simulink model "simulation_file"  (R2023b)
settings: Solver=FixedStepAuto  StartTime=0.0  StopTime=16  FixedStep=0.001  RelTol=1e-3
InitFcn:
  | importfrankaEmikaPanda
values from neighbouring files (symbols this model uses):
  d_influence = 0.06    [distance_with_linesegments_test.m]    (also in importfrankaEmikaPanda.m; matlab_obstacle_avoidance.m = 0.04)
  d_stop = 0.02    [distance_with_linesegments_test.m]    (also in importfrankaEmikaPanda.m; matlab_obstacle_avoidance.m = 0.01)
  Gripper_orientation = [-pi/4 0 0]    [importfrankaEmikaPanda.m]
  Gripper_position = [0 0 0.103399]    [importfrankaEmikaPanda.m]
  Homejointpositions = [0 ,0, 0, -pi/2, 0, pi/2, pi/4]    [importfrankaEmikaPanda.m]
  jointMaxValues = [2.8973, 1.7628, 2.8973, -0.0698, 2.8973, 3.7525, 2.8973]    [importfrankaEmikaPanda.m]
  jointMinValues = [-2.8973, -1.7628, -2.8973, -3.0718, -2.8973, 0.6500, -2.8973]    [importfrankaEmikaPanda.m]
  jointvelMaxValues = [2.1750 2.1750 2.1750 2.1750 2.6100 2.6100 2.6100]    [importfrankaEmikaPanda.m]
  jointvelMinValues = [-2.1750 -2.1750 -2.1750 -2.1750 -2.6100 -2.6100 -2.6100]    [importfrankaEmikaPanda.m]
  m = sqrt(det(JJt))    [computeManipulabilityJacobian.m]
  maxWaypoints = 20    [createWaypointData.m]    (also in importfrankaEmikaPanda.m)
  mdhparams = [ ... (first row only)    [importfrankaEmikaPanda.m]
  obstacle_sphere_1 = struct(     'type', OBSTACLE_SPHERE,      'center', [0, 0.20, 0.8],      'dimensions', [0.1, 0.1, 0.1],      'orientation', [1, 0, 0, 0],      'axis', 0  )    [importfrankaEmikaPanda.m]    (also in matlab_obstacle_avoidance.m = struct(     'type', OBSTACLE_SPHERE,      'center', [0.5545,)
  orientations = [0     0    0 ... (first row only)    [createWaypointData.m]    (also in importfrankaEmikaPanda.m = orientations'; matlab_obstacle_avoidance.m = orientations')
  ts = 0.01    [createWaypointData.m]    (also in importfrankaEmikaPanda.m = 0.001; matlab_obstacle_avoidance.m = 0.001)
  waypointAccels = zeros(size(waypointVels))    [createWaypointData.m]    (also in importfrankaEmikaPanda.m; matlab_obstacle_avoidance.m)
  waypoints = toolPositionHome' +              [0 0 0 ; 0 0 0 ; 0 0 0 ; 0 0 0 ; 0 0 0]'    [createWaypointData.m]    (also in importfrankaEmikaPanda.m = waypoints'; matlab_obstacle_avoidance.m = waypoints')
  waypointTimes = 0:4:16    [createWaypointData.m]    (also in importfrankaEmikaPanda.m; matlab_obstacle_avoidance.m)
  waypointVels = 0.1 *[ 0  0  0 ... (first row only)    [createWaypointData.m]    (also in importfrankaEmikaPanda.m; matlab_obstacle_avoidance.m)
  X = X + v0(1)    [plotCylinder.m]    (also in plotCylinder_foranimation.m)
  Y = Y + v0(2)    [plotCylinder.m]    (also in plotCylinder_foranimation.m)
  Z = Z + v0(3)    [plotCylinder.m]    (also in plotCylinder_foranimation.m)
undefined symbols (not defined in the file or in its folder): diff
libraries: sm_lib x98, nesl_utility x15, robotmaniplib x11, trajExampleUtils x9, robotcorelib x7
(part 3 of 4)

== system simulation_file/Franka Emika Panda/Franka_Robot/panda_link7 ==
  Inertia : sm_lib/Body Elements/Inertia  InertiaType=Custom  Mass=0  MassUnits=kg  CenterOfMass=[0, 0, 0]  CenterOfMassUnits=m  MomentsOfInertia=[0, 0, 0]  MomentsOfInertiaUnits=kg*m^2  ProductsOfInertia=[0, 0, 0]  ProductsOfInertiaUnits=kg*m^2  GraphicType=None  MarkerShape=Inertia  MarkerSize=20  GraphicVisPropType=SimpleVisualProperties  GraphicDiffuseColor=[0.5 0.5 0.5]  GraphicSpecularColor=[0.5 0.5 0.5 1.0]  GraphicAmbientColor=[0.15 0.15 0.15 1.0]  GraphicEmissiveColor=[0.0 0.0 0.0 1.0]  GraphicShininess=75  GraphicOpacity=1.0
  InertiaOriginTransform : sm_lib/Frames and Transforms/Rigid Transform  TranslationMethod=Cartesian  TranslationStandardOffset=0  TranslationStandardOffsetUnits=m  TranslationStandardAxis=+Z  TranslationCartesianOffset=[0, 0, 0]  TranslationCartesianOffsetUnits=m  TranslationROffset=0  TranslationROffsetUnits=m  TranslationZOffset=0  TranslationZOffsetUnits=m  TranslationThetaOffset=0  TranslationThetaOffsetUnits=deg  RotationMethod=RotationSequence  RotationAngleUnits=deg  RotationStandardAxis=+Z  RotationAngle=0.0  RotationArbitraryAxis=[0 0 1]  FollAlignAxisA=+X  BaseAlignAxisA=+Y  FollAlignAxisB=+Y  BaseAlignAxisB=+Z  RotationSequenceAxes=BaseAxes  RotationSequence=XYZ  RotationSequenceAngles=[0, 0, 0]  RotationSequenceAnglesUnits=rad  RotationMatrix=[1 0 0; 0 1 0; 0 0 1]  Quaternion=[1 0 0 0]
  ReferenceFrame : sm_lib/Frames and Transforms/Reference Frame
  Visual : sm_lib/Body Elements/File Solid  ExtGeomFileName=/home/shobhit/Documents/MATLAB/SupportPackages/R2023b/toolbox/robotics/supportpackages/robotlibrary/Robots/franka_description/meshes/visual/link7.stl  UnitType=Custom  ExtGeomFileUnits=m  StepReaderType=HEX  ExportConvexHullGeometry=off  InertiaType=Custom  Mass=0  MassUnits=kg  CenterOfMass=[0, 0, 0]  CenterOfMassUnits=m  MomentsOfInertia=[0, 0, 0]  MomentsOfInertiaUnits=kg*m^2  ProductsOfInertia=[0, 0, 0]  ProductsOfInertiaUnits=kg*m^2  BasedOnType=DensityFromFile  Density=1000  DensityUnits=kg/m^3  DoExposeReferenceFrame=on  SerializedFrames=<Frames/>  GraphicType=FromGeometry  MarkerShape=Sphere  MarkerSize=10  GraphicVisPropType=SimpleVisualProperties  GraphicDiffuseColor=[0.5, 0.5, 0.5]  GraphicSpecularColor=[0.5 0.5 0.5 1.0]  GraphicAmbientColor=[0.15 0.15 0.15 1.0]  GraphicEmissiveColor=[0.0 0.0 0.0 1.0]  GraphicShininess=75  GraphicOpacity=1
  VisualOriginTransform : sm_lib/Frames and Transforms/Rigid Transform  TranslationMethod=Cartesian  TranslationStandardOffset=0  TranslationStandardOffsetUnits=m  TranslationStandardAxis=+Z  TranslationCartesianOffset=[0, 0, 0]  TranslationCartesianOffsetUnits=m  TranslationROffset=0  TranslationROffsetUnits=m  TranslationZOffset=0  TranslationZOffsetUnits=m  TranslationThetaOffset=0  TranslationThetaOffsetUnits=deg  RotationMethod=RotationSequence  RotationAngleUnits=deg  RotationStandardAxis=+Z  RotationAngle=0.0  RotationArbitraryAxis=[0 0 1]  FollAlignAxisA=+X  BaseAlignAxisA=+Y  FollAlignAxisB=+Y  BaseAlignAxisB=+Z  RotationSequenceAxes=BaseAxes  RotationSequence=XYZ  RotationSequenceAngles=[0, 0, 0]  RotationSequenceAnglesUnits=rad  RotationMatrix=[1 0 0; 0 1 0; 0 0 1]  Quaternion=[1 0 0 0]
  panda_joint7_AxisInvTransform : sm_lib/Frames and Transforms/Rigid Transform  TranslationMethod=Cartesian  TranslationStandardOffset=0  TranslationStandardOffsetUnits=m  TranslationStandardAxis=+Z  TranslationCartesianOffset=[0, 0, 0]  TranslationCartesianOffsetUnits=m  TranslationROffset=0  TranslationROffsetUnits=m  TranslationZOffset=0  TranslationZOffsetUnits=m  TranslationThetaOffset=0  TranslationThetaOffsetUnits=deg  RotationMethod=ArbitraryAxis  RotationAngleUnits=rad  RotationStandardAxis=+Z  RotationAngle=0  RotationArbitraryAxis=[1, 0, 0]  FollAlignAxisA=+X  BaseAlignAxisA=+Y  FollAlignAxisB=+Y  BaseAlignAxisB=+Z  RotationSequenceAxes=FollowerAxes  RotationSequence=XYX  RotationSequenceAngles=[0 0 0]  RotationSequenceAnglesUnits=deg  RotationMatrix=[1 0 0; 0 1 0; 0 0 1]  Quaternion=[1 0 0 0]
  panda_joint8_OriginTransform : sm_lib/Frames and Transforms/Rigid Transform  TranslationMethod=Cartesian  TranslationStandardOffset=0  TranslationStandardOffsetUnits=m  TranslationStandardAxis=+Z  TranslationCartesianOffset=[0, 0, 0.107]  TranslationCartesianOffsetUnits=m  TranslationROffset=0  TranslationROffsetUnits=m  TranslationZOffset=0  TranslationZOffsetUnits=m  TranslationThetaOffset=0  TranslationThetaOffsetUnits=deg  RotationMethod=RotationSequence  RotationAngleUnits=deg  RotationStandardAxis=+Z  RotationAngle=0.0  RotationArbitraryAxis=[0 0 1]  FollAlignAxisA=+X  BaseAlignAxisA=+Y  FollAlignAxisB=+Y  BaseAlignAxisB=+Z  RotationSequenceAxes=BaseAxes  RotationSequence=XYZ  RotationSequenceAngles=[0, 0, 0]  RotationSequenceAnglesUnits=rad  RotationMatrix=[1 0 0; 0 1 0; 0 0 1]  Quaternion=[1 0 0 0]
  F : PMIOPort  Side=Left
  F1 : PMIOPort  Port=2  Side=Right
  connections:
  Inertia/RConn1 -- InertiaOriginTransform/RConn1
  ReferenceFrame/RConn1 -- InertiaOriginTransform/LConn1 -- panda_joint7_AxisInvTransform/LConn1 -- panda_joint8_OriginTransform/LConn1 -- VisualOriginTransform/LConn1
  Visual/RConn1 -- VisualOriginTransform/RConn1
  panda_joint7_AxisInvTransform/RConn1 -- F/RConn1
  panda_joint8_OriginTransform/RConn1 -- F1/RConn1

== system simulation_file/Franka Emika Panda/Franka_Robot/panda_link8 ==
  Inertia : sm_lib/Body Elements/Inertia  InertiaType=Custom  Mass=0  MassUnits=kg  CenterOfMass=[0, 0, 0]  CenterOfMassUnits=m  MomentsOfInertia=[0, 0, 0]  MomentsOfInertiaUnits=kg*m^2  ProductsOfInertia=[0, 0, 0]  ProductsOfInertiaUnits=kg*m^2  GraphicType=None  MarkerShape=Inertia  MarkerSize=20  GraphicVisPropType=SimpleVisualProperties  GraphicDiffuseColor=[0.5 0.5 0.5]  GraphicSpecularColor=[0.5 0.5 0.5 1.0]  GraphicAmbientColor=[0.15 0.15 0.15 1.0]  GraphicEmissiveColor=[0.0 0.0 0.0 1.0]  GraphicShininess=75  GraphicOpacity=1.0
  InertiaOriginTransform : sm_lib/Frames and Transforms/Rigid Transform  TranslationMethod=Cartesian  TranslationStandardOffset=0  TranslationStandardOffsetUnits=m  TranslationStandardAxis=+Z  TranslationCartesianOffset=[0, 0, 0]  TranslationCartesianOffsetUnits=m  TranslationROffset=0  TranslationROffsetUnits=m  TranslationZOffset=0  TranslationZOffsetUnits=m  TranslationThetaOffset=0  TranslationThetaOffsetUnits=deg  RotationMethod=RotationSequence  RotationAngleUnits=deg  RotationStandardAxis=+Z  RotationAngle=0.0  RotationArbitraryAxis=[0 0 1]  FollAlignAxisA=+X  BaseAlignAxisA=+Y  FollAlignAxisB=+Y  BaseAlignAxisB=+Z  RotationSequenceAxes=BaseAxes  RotationSequence=XYZ  RotationSequenceAngles=[0, 0, 0]  RotationSequenceAnglesUnits=rad  RotationMatrix=[1 0 0; 0 1 0; 0 0 1]  Quaternion=[1 0 0 0]
  ReferenceFrame : sm_lib/Frames and Transforms/Reference Frame
  panda_hand_joint_OriginTransform : sm_lib/Frames and Transforms/Rigid Transform  TranslationMethod=Cartesian  TranslationStandardOffset=0  TranslationStandardOffsetUnits=m  TranslationStandardAxis=+Z  TranslationCartesianOffset=[0, 0, 0]  TranslationCartesianOffsetUnits=m  TranslationROffset=0  TranslationROffsetUnits=m  TranslationZOffset=0  TranslationZOffsetUnits=m  TranslationThetaOffset=0  TranslationThetaOffsetUnits=deg  RotationMethod=RotationSequence  RotationAngleUnits=deg  RotationStandardAxis=+Z  RotationAngle=0.0  RotationArbitraryAxis=[0 0 1]  FollAlignAxisA=+X  BaseAlignAxisA=+Y  FollAlignAxisB=+Y  BaseAlignAxisB=+Z  RotationSequenceAxes=BaseAxes  RotationSequence=XYZ  RotationSequenceAngles=[0, 0, -0.785398163397]  RotationSequenceAnglesUnits=rad  RotationMatrix=[1 0 0; 0 1 0; 0 0 1]  Quaternion=[1 0 0 0]
  F : PMIOPort  Side=Left
  F1 : PMIOPort  Port=2  Side=Right
  connections:
  Inertia/RConn1 -- InertiaOriginTransform/RConn1
  ReferenceFrame/RConn1 -- InertiaOriginTransform/LConn1 -- panda_hand_joint_OriginTransform/LConn1 -- F/RConn1
  panda_hand_joint_OriginTransform/RConn1 -- F1/RConn1

== system simulation_file/Franka Emika Panda/Franka_Robot/panda_rightfinger ==
  Inertia : sm_lib/Body Elements/Inertia  InertiaType=Custom  Mass=0  MassUnits=kg  CenterOfMass=[0, 0, 0]  CenterOfMassUnits=m  MomentsOfInertia=[0, 0, 0]  MomentsOfInertiaUnits=kg*m^2  ProductsOfInertia=[0, 0, 0]  ProductsOfInertiaUnits=kg*m^2  GraphicType=None  MarkerShape=Inertia  MarkerSize=20  GraphicVisPropType=SimpleVisualProperties  GraphicDiffuseColor=[0.5 0.5 0.5]  GraphicSpecularColor=[0.5 0.5 0.5 1.0]  GraphicAmbientColor=[0.15 0.15 0.15 1.0]  GraphicEmissiveColor=[0.0 0.0 0.0 1.0]  GraphicShininess=75  GraphicOpacity=1.0
  InertiaOriginTransform : sm_lib/Frames and Transforms/Rigid Transform  TranslationMethod=Cartesian  TranslationStandardOffset=0  TranslationStandardOffsetUnits=m  TranslationStandardAxis=+Z  TranslationCartesianOffset=[0, 0, 0]  TranslationCartesianOffsetUnits=m  TranslationROffset=0  TranslationROffsetUnits=m  TranslationZOffset=0  TranslationZOffsetUnits=m  TranslationThetaOffset=0  TranslationThetaOffsetUnits=deg  RotationMethod=RotationSequence  RotationAngleUnits=deg  RotationStandardAxis=+Z  RotationAngle=0.0  RotationArbitraryAxis=[0 0 1]  FollAlignAxisA=+X  BaseAlignAxisA=+Y  FollAlignAxisB=+Y  BaseAlignAxisB=+Z  RotationSequenceAxes=BaseAxes  RotationSequence=XYZ  RotationSequenceAngles=[0, 0, 0]  RotationSequenceAnglesUnits=rad  RotationMatrix=[1 0 0; 0 1 0; 0 0 1]  Quaternion=[1 0 0 0]
  ReferenceFrame : sm_lib/Frames and Transforms/Reference Frame
  Visual : sm_lib/Body Elements/File Solid  ExtGeomFileName=/home/shobhit/Documents/MATLAB/SupportPackages/R2023b/toolbox/robotics/supportpackages/robotlibrary/Robots/franka_description/meshes/visual/finger.stl  UnitType=Custom  ExtGeomFileUnits=m  StepReaderType=HEX  ExportConvexHullGeometry=off  InertiaType=Custom  Mass=0  MassUnits=kg  CenterOfMass=[0, 0, 0]  CenterOfMassUnits=m  MomentsOfInertia=[0, 0, 0]  MomentsOfInertiaUnits=kg*m^2  ProductsOfInertia=[0, 0, 0]  ProductsOfInertiaUnits=kg*m^2  BasedOnType=DensityFromFile  Density=1000  DensityUnits=kg/m^3  DoExposeReferenceFrame=on  SerializedFrames=<Frames/>  GraphicType=FromGeometry  MarkerShape=Sphere  MarkerSize=10  GraphicVisPropType=SimpleVisualProperties  GraphicDiffuseColor=[0.5, 0.5, 0.5]  GraphicSpecularColor=[0.5 0.5 0.5 1.0]  GraphicAmbientColor=[0.15 0.15 0.15 1.0]  GraphicEmissiveColor=[0.0 0.0 0.0 1.0]  GraphicShininess=75  GraphicOpacity=1
  VisualOriginTransform : sm_lib/Frames and Transforms/Rigid Transform  TranslationMethod=Cartesian  TranslationStandardOffset=0  TranslationStandardOffsetUnits=m  TranslationStandardAxis=+Z  TranslationCartesianOffset=[0, 0, 0]  TranslationCartesianOffsetUnits=m  TranslationROffset=0  TranslationROffsetUnits=m  TranslationZOffset=0  TranslationZOffsetUnits=m  TranslationThetaOffset=0  TranslationThetaOffsetUnits=deg  RotationMethod=RotationSequence  RotationAngleUnits=deg  RotationStandardAxis=+Z  RotationAngle=0.0  RotationArbitraryAxis=[0 0 1]  FollAlignAxisA=+X  BaseAlignAxisA=+Y  FollAlignAxisB=+Y  BaseAlignAxisB=+Z  RotationSequenceAxes=BaseAxes  RotationSequence=XYZ  RotationSequenceAngles=[0, 0, -3.141592653589587]  RotationSequenceAnglesUnits=rad  RotationMatrix=[1 0 0; 0 1 0; 0 0 1]  Quaternion=[1 0 0 0]
  panda_finger_joint2_AxisInvTransform : sm_lib/Frames and Transforms/Rigid Transform  TranslationMethod=Cartesian  TranslationStandardOffset=0  TranslationStandardOffsetUnits=m  TranslationStandardAxis=+Z  TranslationCartesianOffset=[0, 0, 0]  TranslationCartesianOffsetUnits=m  TranslationROffset=0  TranslationROffsetUnits=m  TranslationZOffset=0  TranslationZOffsetUnits=m  TranslationThetaOffset=0  TranslationThetaOffsetUnits=deg  RotationMethod=ArbitraryAxis  RotationAngleUnits=rad  RotationStandardAxis=+Z  RotationAngle=1.570796326794897  RotationArbitraryAxis=[1, 0, 0]  FollAlignAxisA=+X  BaseAlignAxisA=+Y  FollAlignAxisB=+Y  BaseAlignAxisB=+Z  RotationSequenceAxes=FollowerAxes  RotationSequence=XYX  RotationSequenceAngles=[0 0 0]  RotationSequenceAnglesUnits=deg  RotationMatrix=[1 0 0; 0 1 0; 0 0 1]  Quaternion=[1 0 0 0]
  F : PMIOPort  Side=Left
  connections:
  Inertia/RConn1 -- InertiaOriginTransform/RConn1
  ReferenceFrame/RConn1 -- InertiaOriginTransform/LConn1 -- VisualOriginTransform/LConn1 -- panda_finger_joint2_AxisInvTransform/LConn1
  Visual/RConn1 -- VisualOriginTransform/RConn1
  panda_finger_joint2_AxisInvTransform/RConn1 -- F/RConn1

== system simulation_file/Trajectory Generation/Rotation Trajectory/Extract Trajectory Segment ==
  segIdx : Inport
  waypointTimes : Inport  Port=2
  orientations : Inport  Port=3
  Enable : EnablePort  PropagateVarSize=During execution
  MATLAB Function : MATLAB Function  Commented=on  TreatAsAtomicUnit=on
  MATLAB Function1 : MATLAB Function  TreatAsAtomicUnit=on
  q0 : Outport  VectorParamsAs1DForOutWhenUnconnected=off
  qf : Outport  Port=2  VectorParamsAs1DForOutWhenUnconnected=off
  timeInterval : Outport  Port=3  VectorParamsAs1DForOutWhenUnconnected=off
  wires:
  segIdx/1 -> MATLAB Function1/1(segIdx)
  MATLAB Function1/1(q0) -> q0/1
  MATLAB Function1/3(timeInterval) -> timeInterval/1
  orientations/1 -> MATLAB Function1/3(orientations)
  MATLAB Function1/2(qf) -> qf/1
  waypointTimes/1 -> MATLAB Function1/2(waypointTimes)

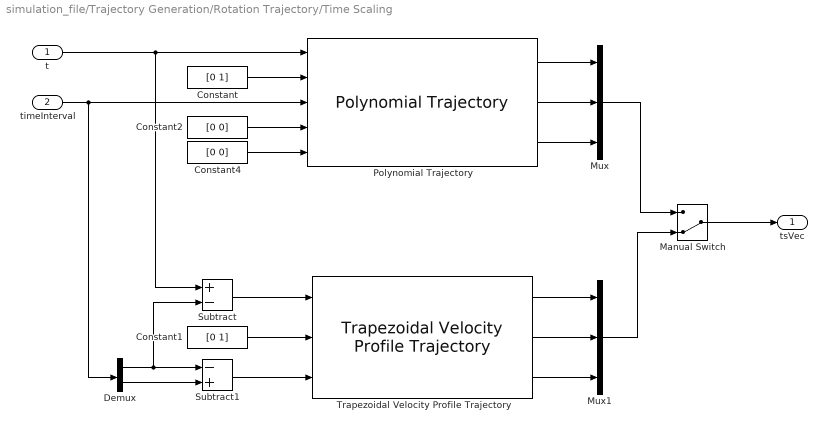
== system simulation_file/Trajectory Generation/Rotation Trajectory/Time Scaling ==
  t : Inport
  timeInterval : Inport  Port=2
  Constant : Constant  Value=[0 1]  VectorParams1D=off
  Constant1 : Constant  Value=[0 1]  VectorParams1D=off
  Constant2 : Constant  Value=[0 0]  VectorParams1D=off
  Constant4 : Constant  Value=[0 0]  VectorParams1D=off
  Demux : Demux  Outputs=2
  Manual Switch : ManualSwitch  CurrentSetting=0
  Mux : Mux  Inputs=3
  Mux1 : Mux  Inputs=3
  Polynomial Trajectory : robotcorelib/Polynomial Trajectory  WaypointSource=External  Waypoints=[ 0, 2, 1, 5, 0; -1, 3, 1, 4, 4 ]  TimePoints=[ 0, 1, 2, 3, 4 ]  TimeInterval=[ 1, 4 ]  Method=Quintic Polynomial  ParameterSource=External  VelocityBoundaryCondition=zeros( 2, 5 )  AccelerationBoundaryCondition=zeros( 2, 5 )  SimulateUsing=Interpreted execution
  Subtract : Sum  Inputs=+-
  Subtract1 : Sum  Inputs=-+
  Trapezoidal Velocity Profile Trajectory : robotcorelib/Trapezoidal Velocity Profile Trajectory  WaypointSource=External  Waypoints=[ 0, -0.5, -1; 0, 0.5, 1 ]  NumParams=1  Parameter1=End Time  Parameter2=End Time  ParameterSource=External  PeakVelocity=[ 2; 2 ]  Acceleration=[ 1; 2 ]  EndTime=[ 1; 1 ]  AccelTime=[ 1; 2 ]  SimulateUsing=Interpreted execution
  tsVec : Outport  VectorParamsAs1DForOutWhenUnconnected=off
  wires:
  Manual Switch/1 -> tsVec/1
  Polynomial Trajectory/3 -> Mux/3
  Polynomial Trajectory/1 -> Mux/1
  Constant/1 -> Polynomial Trajectory/2
  Constant4/1 -> Polynomial Trajectory/5
  Constant2/1 -> Polynomial Trajectory/4
  Polynomial Trajectory/2 -> Mux/2
  t/1 -> Polynomial Trajectory/1, Subtract/1
  Mux/1 -> Manual Switch/1
  Trapezoidal Velocity Profile Trajectory/1 -> Mux1/1
  Trapezoidal Velocity Profile Trajectory/2 -> Mux1/2
  Trapezoidal Velocity Profile Trajectory/3 -> Mux1/3
  Mux1/1 -> Manual Switch/2
  Constant1/1 -> Trapezoidal Velocity Profile Trajectory/2
  timeInterval/1 -> Demux/1, Polynomial Trajectory/3
  Subtract1/1 -> Trapezoidal Velocity Profile Trajectory/3
  Demux/1 -> Subtract/2, Subtract1/1
  Subtract/1 -> Trapezoidal Velocity Profile Trajectory/1
  Demux/2 -> Subtract1/2

== matlab function simulation_file/MATLAB Function5 ==
  data: u input; y output
function y = fcn(u)
otfunction y = fcn(u)
y = det()
y = u;

== matlab function simulation_file/MATLAB Function1 ==
  data: jointvalues input; newjointvalues_withgripper output
function newjointvalues_withgripper = concatenatejoints(jointvalues)
newjointvalues_withgripper = zeros(9,1);
newjointvalues_withgripper(1:7) = jointvalues; 

end

== matlab function simulation_file/Manual INVERSE KINEMATICS BlOCK/Constrained_Inverse_Kinematics/MATLAB Function1 ==
  settings: updateMethod=DISCRETE
  data: joint_values input; optimal_joint_velocity output; jacobi input; weights input; xd_eff_vel input; jointminvalues input; jointmaxvalues input; joint_min_vel input; joint_max_vel input; current_joint_vel input; J_g input; b_g input
function optimal_joint_velocity = inverse_kinematics_constraints(joint_values,jacobi,weights,xd_eff_vel,jointminvalues,jointmaxvalues,joint_min_vel,joint_max_vel,current_joint_vel,J_g,b_g)
persistent starting_joint_vel is_first_step

  
% Initialize 'starting_joint_vel' if it's the first execution or if it's undefined
if isempty(is_first_step) || isempty(starting_joint_vel)
    is_first_step = true;
    starting_joint_vel = zeros(7,1); % Default initialization
end

% Then, check if it's the first execution step to perform any first-time setup
if is_first_step
    is_first_step = false; % Ensure this block won't execute again
    % No need to set 'starting_joint_vel' here again if it's already set above
end
jointminvalues = jointminvalues';
jointmaxvalues = jointmaxvalues';
joint_min_vel = joint_min_vel';
joint_max_vel = joint_max_vel';


delta = weights(1);
alpha = weights(2);
beta = weights(3);
omega = weights(4);


%sg = 1;
objective = @(q_vel) omega  * (norm(q_vel, Inf)^2) / 2 + ... % infinity norm term
                       delta * (norm(q_vel, 2)^2 )/ 2 + ... % two-norm term
                       alpha * sum((q_vel - starting_joint_vel).^2) + ...
                       beta * 1/(1 + smin(jacobi)) ; % additional term from Eq. (2.17)

% sum((q_vel - current_joint_vel).^2) 
% objective = @(q_vel) (1-delta-alpha-beta)  * (norm(q_vel, Inf)^2) / 2 + ... % infinity norm term
%                        delta * (norm(q_vel, 2)^2 )/ 2 + ... % two-norm term
%                        alpha * ((q_vel * eye(length(q_vel))*q_vel') + 2* sg * q_vel  ) / 2 + ...
%                        beta * 1/(1 + sqrt(det(jacobi' * jacobi))) ; % additional term from Eq. (2.17)
% A = J_g; b = b_g;
A = [];  b = []; % No linear inequality constraints
Aeq = jacobi; beq = xd_eff_vel; % No linear equality constraints

%gamma is a positive parameter used to control the range of q_vel
gamma = 0.5;
% lb = max(gamma*(jointminvalues - joint_values),joint_min_vel); % Lower bound from Eq. (2.14)
% ub = min(gamma*(jointmaxvalues - joint_values),joint_max_vel); % Upper bound from Eq. (2.15)
lb = max(gamma .* (jointminvalues - joint_values), joint_min_vel); % Element-wise max
ub = min(gamma .* (jointmaxvalues - joint_values), joint_max_vel); % Element-wise min

% Define the nonlinear constraint function
% nonlcon = @(theta) deal(... % Use 'deal' to output both C and Ceq for fmincon
%     Jc(theta) - bc, ... % Inequality constraints from Eq. (2.13)
%     Je(theta) - re ... % Equality constraints from Eq. (2.12)
% );

% Set up optimization options (optional)
%options = optimoptions('fmincon', 'Algorithm', 'interior-point', ... % Choose an algorithm
                       % 'Display', 'iter', ... % Display iterations
                       % 'MaxIterations', 1000, ... % Maximum number of iterations
                       % 'ConstraintTolerance', 1e-6); % Constraint tolerance
options = optimoptions('fmincon','Algorithm','sqp');
% Initial guess for theta
q_vel_initial_guess = starting_joint_vel;  % You need to provide an initial guess
 
% Run the optimization
[q_vel_opt, fval,Exit_Flag] = fmincon(objective, q_vel_initial_guess, A, b, Aeq, beq, lb, ub, [], options);

% Output the results
disp('Optimal joint velocity:');
disp(q_vel_opt);
disp('Objective function value at optimal joint velocity:');
disp(fval);
disp('exit Flag: ')
disp(Exit_Flag);
starting_joint_vel = q_vel_opt;


optimal_joint_velocity = q_vel_opt;
end

== matlab function simulation_file/Manual INVERSE KINEMATICS BlOCK/Constrained_Inverse_Kinematics/MATLAB Function2 ==
  data: J input; jacobi output
function jacobi  = rearrangejacobi(J)
%use only if using the toolbox jacobi is used as input


J_i = zeros(6,7);
J_i(1:3,1:end) = J(4:end,1:end);
J_i(4:end,1:end) = J(1:3,1:end);
jacobi = J_i;


end

== matlab function simulation_file/MATLAB Function ==
  settings: updateMethod=DISCRETE
  data: jointValues input
function storeJointValues(jointValues)
    % Define a persistent variable to store joint angles over time
    persistent jointAnglesMatrix;
    if isempty(jointAnglesMatrix)
        % Initialize the persistent variable with an empty matrix
        jointAnglesMatrix = [];
    end

    % Concatenate the new joint values to the matrix
    jointAnglesMatrix = [jointAnglesMatrix; jointValues'];

    % Use a cleanup object to save data when the simulation is stopped
    cleanupObj = onCleanup(@()assignin('base', 'jointAnglesMatrix', jointAnglesMatrix));
end

== matlab function simulation_file/Manual INVERSE KINEMATICS BlOCK/Constrained_Inverse_Kinematics/MATLAB Function3 ==
  settings: updateMethod=DISCRETE
  data: robot input; joint_values input; optimal_joint_velocity output; jacobi input; weights input; xd_eff_vel input; jointminvalues input; jointmaxvalues input; joint_min_vel input; joint_max_vel input; current_joint_vel input
function optimal_joint_velocity = obstacle_avoidance_with_inverse_kinematics(robot,joint_values,jacobi,weights,xd_eff_vel,jointminvalues,jointmaxvalues,joint_min_vel,joint_max_vel,current_joint_vel)
persistent starting_joint_vel is_first_step

  
% Initialize 'starting_joint_vel' if it's the first execution or if it's undefined
if isempty(is_first_step) || isempty(starting_joint_vel)
    is_first_step = true;
    starting_joint_vel = zeros(1,7); % Default initialization
end

% Then, check if it's the first execution step to perform any first-time setup
if is_first_step
    is_first_step = false; % Ensure this block won't execute again
    % No need to set 'starting_joint_vel' here again if it's already set above
end

delta = weights(1);
alpha = weights(2);
beta = weights(3);
omega = weights(4);


%sg = 1;
objective = @(q_vel) omega  * (norm(q_vel, Inf)^2) / 2 + ... % infinity norm term
                       delta * (norm(q_vel, 2)^2 )/ 2 + ... % two-norm term
                       alpha * sum((q_vel - starting_joint_vel).^2) + ...
                       beta * 1/(1 + smin(jacobi)) ; % additional term from Eq. (2.17)

% sum((q_vel - current_joint_vel).^2) 
% objective = @(q_vel) (1-delta-alpha-beta)  * (norm(q_vel, Inf)^2) / 2 + ... % infinity norm term
%                        delta * (norm(q_vel, 2)^2 )/ 2 + ... % two-norm term
%                        alpha * ((q_vel * eye(length(q_vel))*q_vel') + 2* sg * q_vel  ) / 2 + ...
%                        beta * 1/(1 + sqrt(det(jacobi' * jacobi))) ; % additional term from Eq. (2.17)
A = []; b = []; % No linear inequality constraints
Aeq = jacobi; beq = xd_eff_vel; % No linear equality constraints

%gamma is a positive parameter used to control the range of q_vel
gamma = 0.5
% lb = max(gamma*(jointminvalues - joint_values),joint_min_vel); % Lower bound from Eq. (2.14)
% ub = min(gamma*(jointmaxvalues - joint_values),joint_max_vel); % Upper bound from Eq. (2.15)
lb = max(gamma .* (jointminvalues - joint_values), joint_min_vel); % Element-wise max
ub = min(gamma .* (jointmaxvalues - joint_values), joint_max_vel); % Element-wise min

% Define the nonlinear constraint function
% nonlcon = @(theta) deal(... % Use 'deal' to output both C and Ceq for fmincon
%     Jc(theta) - bc, ... % Inequality constraints from Eq. (2.13)
%     Je(theta) - re ... % Equality constraints from Eq. (2.12)
% );

% Set up optimization options (optional)
%options = optimoptions('fmincon', 'Algorithm', 'interior-point', ... % Choose an algorithm
                       % 'Display', 'iter', ... % Display iterations
                       % 'MaxIterations', 1000, ... % Maximum number of iterations
                       % 'ConstraintTolerance', 1e-6); % Constraint tolerance
options = optimoptions('fmincon','Algorithm','sqp');
% Initial guess for theta
q_vel_initial_guess = starting_joint_vel;  % You need to provide an initial guess
 
% Run the optimization
[q_vel_opt, fval,Exit_Flag] = fmincon(objective, q_vel_initial_guess, A, b, Aeq, beq, lb, ub, [], options);

% Output the results
disp('Optimal joint velocity:');
disp(q_vel_opt);
disp('Objective function value at optimal joint velocity:');
disp(fval);
disp('exit Flag: ')
disp(Exit_Flag);
starting_joint_vel = q_vel_opt;


optimal_joint_velocity = q_vel_opt;
end

== matlab function simulation_file/Manual INVERSE KINEMATICS BlOCK/Obstacle_Avoidance_dynamic_inequality ==
  data: obstacles input; jointAngles input; mdhparams input; J_g output; radius_of_linesegments input; d_influence input; d_stop input; b_g output; Homejointpositions input; jointMinValues input; jointMaxValues input; Gripper_position input; Gripper_orientation input
function [J_g,b_g] = obstacle_avoidance_equation(obstacles,jointAngles,mdhparams,radius_of_linesegments,d_influence,d_stop,Homejointpositions,jointMinValues,jointMaxValues,Gripper_position,Gripper_orientation)
%run before this importfrankaemika
%robot = frankarobot_mdh;
%radius for each link
radius = radius_of_linesegments;
%d_influence = 0.06;
%d_stop = 0.02;
%jointAngles = Homejointpositions;

% Define persistent variables to store the critical points and related data
    persistent criticalPoints robot
if isempty(robot)
robot = give_robot(mdhparams,Homejointpositions,jointMinValues,jointMaxValues,Gripper_position,Gripper_orientation);
end
    
    % Initialize the persistent variables if they are empty (first run)
    numLinks = length(mdhparams); % Number of line segments
    numObstacles = length(obstacles); % Number of obstacles
    number_of_joints = length(jointAngles);
    %default_vector = [NaN NaN NaN];
    if isempty(criticalPoints)
               criticalPoints = repmat(struct(...
           'roc_A',nan(1,3), ...
            'roc_D',nan(1,3), ...
            'has_criticalpoints_A', false, ...
            'has_criticalpoints_D', false, ...
            'jacobi_dist_max_A', nan(3,number_of_joints), ...
            'jacobi_dist_max_D', nan(3,number_of_joints), ...
            'jointAngles_critical_A', nan(1,number_of_joints), ...
            'jointAngles_critical_D', nan(1,number_of_joints), ...
            'jacobi_distance_A', nan(3,number_of_joints), ...
            'jacobi_distance_D', nan(3,number_of_joints), ...
            'distance', NaN,   ...
            'reletive_distance', [] ...
        ), numLinks, numObstacles);
    end


%create line swept spheres of robot links with help of modiefied dh
%parameters and current joint configuration with 
linesegments = createLineSegments(mdhparams,robot,radius,jointAngles);
% roc = 0;
% for l=1:length(obstacles)
%     for i=1:length(linesegments)
%         if(isempty(linesegments(i).has_criticalpoints_A(l)))
%             linesegments(i).has_criticalpoints_A(l) = false;
%         end
%         if (isempty(linesegments(i).has_criticalpoints_D(l)))
%             linesegments(i).has_criticalpoints_D(l) = false;
%         end
%         linesegments(i).jacobi_distance_A(l) = [];
%         linesegments(i).jacobi_distance_D(l) = [];
% 
%     end
% end


for l = 1:length(obstacles)

    for i = 1:length(linesegments)
        %Calculate distance for a and dsegments
        criticalPoints(i,l).jacobi_distance_A = nan(3,number_of_joints);
        criticalPoints(i,l).jacobi_distance_D = nan(3,number_of_joints);
        
            if criticalPoints(i,l).has_criticalpoints_A && ~any(isnan(criticalPoints(i,l).roc_A)) %&& norm(linesegments(i).roc_A) <= d_influence
                T_Ca = getTransform(robot,jointAngles,sprintf('Critical_Point_Link_A_%d%d', int32(i), int32(l)),'base');
                position_ca = T_Ca(1:3,4);
                roc = position_ca-(obstacles(l).center)' ;
                roc_normalised = roc ./ norm(roc);
                dist_roc = norm(roc) - obstacles(l).dimensions(1) - linesegments(i).radius;
                dist_crit_a = dist_roc * roc_normalised;
                 J = rearrangejacobi(geometricJacobian(robot,jointAngles,sprintf('Critical_Point_Link_A_%d%d', int32(i), int32(l))),length(jointAngles));
                 %escape velocity 
                 criticalPoints(i,l).jacobi_distance_A = [-dist_crit_a(1) * J(1,1:end); -dist_crit_a(2) * J(2,1:end); -dist_crit_a(3) * J(3,1:end)];
                 criticalPoints(i,l).distance = dist_roc; 
             
                 criticalPoints(i,l).roc_A = dist_crit_a';
            end
                 %Calculate distance between 0 and Critcal Point 

             if criticalPoints(i,l).has_criticalpoints_D && ~any(isnan(criticalPoints(i,l).roc_D)) %&& norm(linesegments(i).roc_D) <= d_influence
                 T_Cd = getTransform(robot,jointAngles,sprintf('Critical_Point_Link_D_%d%d', int32(i), int32(l)),'base');
                position_cd = T_Cd(1:3,4);
                roc = position_cd-(obstacles(l).center)' ;
                roc_normalised = roc ./ norm(roc);
                dist_roc = norm(roc) - obstacles(l).dimensions(1) - linesegments(i).radius;
                dist_crit_d = dist_roc * roc_normalised;
                 J = rearrangejacobi(geometricJacobian(robot,jointAngles,sprintf('Critical_Point_Link_D_%d%d', int32(i), int32(l))),length(jointAngles));
                  %escape velocity  
                 criticalPoints(i,l).jacobi_distance_D = [-dist_crit_d(1) * J(1,1:end); -dist_crit_d(2) * J(2,1:end);-dist_crit_d(3) * J(3,1:end)];
                  criticalPoints(i,l).distance = dist_roc; 
                 criticalPoints(i,l).roc_D = dist_crit_d';
             end 

        if ~any(isnan(linesegments(i).aSegmentV0)) && any(isnan(criticalPoints(i,l).roc_A)) && ~(criticalPoints(i,l).has_criticalpoints_A)
            %calculate critical point only if out of critical zone
            %if r_oc  > d_influence

                %at each link at kacobis to linesegement struct
                [s_range_A,dist_A,distA_v1,distA_v0] =  calculate_distance_lss_pss(linesegments(i).aSegmentV0,linesegments(i).aSegmentV1, ...
                    linesegments(i).radius,obstacles(l).center,obstacles(l).dimensions(1));
                if norm(dist_A) <= d_influence
                 critcal_point_inworldframe_A = linesegments(i).aSegmentV0 + s_range_A * (linesegments(i).aSegmentV1 - linesegments(i).aSegmentV0); 
                   
                 %dist betweeb i-1 link origin and critical point on that segmentA on i link
                 T_basetolink = getTransform(robot,jointAngles,'base',sprintf('robot_link%d',int32(i-1))); 
                 if i == 1 
                     T_basetolink = eye(4);
                 end
                 relative_distance_a_vo_toCrit = relative_distance_in_linkframe(T_basetolink,critcal_point_inworldframe_A);   
                 
                  
                       
                    %critical point a_i w.r.t i-1 frame
                    body_critical_A = generate_Criticalbody(sprintf('Critical_Point_Link_A_%d%d', int32(i), int32(l)),sprintf('Critical_Joint_Frame_A_%d%d', int32(i), int32(l)),relative_distance_a_vo_toCrit);
                    if i == 1
                    %add body to base link 
                     addBody(robot,body_critical_A,"base");
                    end 
                     addBody(robot,body_critical_A,sprintf('robot_link%d',int32(i-1)));
                     
                     J = rearrangejacobi(geometricJacobian(robot,jointAngles,sprintf('Critical_Point_Link_A_%d%d', int32(i), int32(l))),length(jointAngles));
                      criticalPoints(i,l).jacobi_distance_A  = [-dist_A(1)*J(1,1:end);-dist_A(2)*J(2,1:end);-dist_A(3)*J(3,1:end)];

                     criticalPoints(i,l).jacobi_dist_max_A = criticalPoints(i,l).jacobi_distance_A;
                     criticalPoints(i,l).has_criticalpoints_A = true;
                     criticalPoints(i,l).jointAngles_critical_A = jointAngles;
                    
                     criticalPoints(i,l).roc_A = dist_A;
                     criticalPoints(i,l).distance = norm(dist_A);
                end 
                if ~any(isnan(linesegments(i).dSegmentV0)) && any(isnan(criticalPoints(i,l).roc_D)) && ~(criticalPoints(i,l).has_criticalpoints_D)
                
                    [s_range_D,dist_D,distD_v1,distD_v0] =  calculate_distance_lss_pss(linesegments(i).dSegmentV0,linesegments(i).dSegmentV1, ...
                    linesegments(i).radius,obstacles(l).center,obstacles(l).dimensions(1));
                %if dist <= d_influence
                    %when distance less than influence distance of obstacle avoidance
                    %get critical point and jacobi at this avoidance scheme starting phase
                    criticalPoints(i,l).distance = min(norm(dist_A),norm(dist_D));
                    if norm(dist_D) <= d_influence 
                     critcal_point_inworldframe_D = linesegments(i).dSegmentV0 + s_range_D * (linesegments(i).dSegmentV1 - linesegments(i).dSegmentV0);
                    
                  
                   %dist betweeb i-1 link origin and critical point on that segmentD on i link
                   T_basetolink = getTransform(robot,jointAngles,'base',sprintf('robot_link%d',int32(i-1))); 
                    if i == 1 
                     T_basetolink = eye(4);
                    end
                   relative_distance_d_vo_toCrit = relative_distance_in_linkframe(T_basetolink,critcal_point_inworldframe_D);
                  
                    
                    body_critical_D = generate_Criticalbody(sprintf('Critical_Point_Link_D_%d%d', int32(i), int32(l)),sprintf('Critical_Joint_Frame_D_%d%d', int32(i), int32(l)),relative_distance_d_vo_toCrit);
                        if i == 1
    
                            addBody(robot,body_critical_D,"base");
                        end
                       
                     addBody(robot,body_critical_D,sprintf('robot_link%d',int32(i-1)));
                     %Jacobi_max at d = d2 
                     J = rearrangejacobi(geometricJacobian(robot,jointAngles,sprintf('Critical_Point_Link_D_%d%d', int32(i), int32(l))),length(jointAngles));
                     criticalPoints(i,l).jacobi_distance_D = [-dist_D(1)*J(1,1:end);-dist_D(2)*J(2,1:end);-dist_D(3)*J(3,1:end)];

                     criticalPoints(i,l).jacobi_dist_max_D = criticalPoints(i,l).jacobi_distance_D;
                     criticalPoints(i,l).has_criticalpoints_D = true;
                     criticalPoints(i,l).jointAngles_critical_D = jointAngles;
                     
                     criticalPoints(i,l).roc_D = dist_D;
                    end 
                end
                %end
            
        end
        
        if any(isnan(linesegments(i).aSegmentV0)) && ~any(isnan(linesegments(i).dSegmentV0)) && any(isnan(criticalPoints(i,l).roc_D)) && ~(criticalPoints(i,l).has_criticalpoints_D)
           [s_range_D,dist_D,distD_v1,distD_v0] =  calculate_distance_lss_pss(linesegments(i).dSegmentV0,linesegments(i).dSegmentV1, ...
                    linesegments(i).radius,obstacles(l).center,obstacles(l).dimensions(1));
           
           criticalPoints(i,l).distance = norm(dist_D);
           if norm(dist_D) <= d_influence 
                critcal_point_inworldframe_D = linesegments(i).dSegmentV0 + s_range_D * (linesegments(i).dSegmentV1 - linesegments(i).dSegmentV0);
               
                %dist betweeb i-1 link origin and critical point on that segmentD on i link
                   T_basetolink = getTransform(robot,jointAngles,'base',sprintf('robot_link%d',int32(i-1))); 
                    if i == 1 
                     T_basetolink = eye(4);
                    end
                   relative_distance_d_vo_toCrit = relative_distance_in_linkframe(T_basetolink,critcal_point_inworldframe_D);
                
                
            body_critical_D = generate_Criticalbody(sprintf('Critical_Point_Link_D_%d%d', int32(i), int32(l)),sprintf('Critical_Joint_Frame_D_%d%d', int32(i), int32(l)),relative_distance_d_vo_toCrit);
            if i == 1
                %add body to base link
                addBody(robot,body_critical_D,"base");
            end
                     addBody(robot,body_critical_D,sprintf('robot_link%d',int32(i-1)));
           

           %Jacobi_max at d = d2 
           J = rearrangejacobi(geometricJacobian(robot,jointAngles,sprintf('Critical_Point_Link_D_%d%d', int32(i), int32(l))),length(jointAngles));
           criticalPoints(i,l).jacobi_distance_D = [-dist_D(1)*J(1,1:end);-dist_D(2)*J(2,1:end);-dist_D(3)*J(3,1:end)];

           criticalPoints(i,l).jacobi_dist_max_D = criticalPoints(i,l).jacobi_distance_D;
           criticalPoints(i,l).has_criticalpoints_D = true;
           criticalPoints(i,l).jointAngles_critical_D = jointAngles;
           
            criticalPoints(i,l).roc_D = dist_D;
           end 
        end
        
        %Delete Critical Points when out of zone (Cleanup of rigidbody
        %critical points
        if ~any(isnan(criticalPoints(i,l).roc_A)) && norm(criticalPoints(i,l).roc_A) > d_influence && criticalPoints(i,l).has_criticalpoints_A
            removeBody(robot,sprintf('Critical_Point_Link_A_%d%d', int32(i), int32(l)));
            criticalPoints(i,l).has_criticalpoints_A = false ;
            criticalPoints(i,l).roc_A  = nan(1,3);
            criticalPoints(i,l).jacobi_distance_A = nan(3,number_of_joints);
            criticalPoints(i,l).jacobi_dist_max_A = nan(3,number_of_joints);
            criticalPoints(i,l).jointAngles_critical_A = nan(1,number_of_joints);

        end 

          if ~any(isnan(criticalPoints(i,l).roc_D)) && norm(criticalPoints(i,l).roc_D)> d_influence && criticalPoints(i,l).has_criticalpoints_D
            removeBody(robot,sprintf('Critical_Point_Link_D_%d%d', int32(i), int32(l)));
            criticalPoints(i,l).has_criticalpoints_D = false ;
            criticalPoints(i,l).roc_D  = nan(1,3);
            criticalPoints(i,l).jacobi_distance_D = nan(3,number_of_joints);
            criticalPoints(i,l).jacobi_dist_max_D = nan(3,number_of_joints);
            criticalPoints(i,l).jointAngles_critical_D = nan(1,number_of_joints);
          end 

    end

end

% %concatenate all the Jg and b_g after calculation of b_g
% J_g = [];
% b_g = [];
% 
% for l = 1:length(obstacles)
%     for i = 1:length(linesegments)
%         J_g = [J_g; criticalPoints(i,l).jacobi_distance_A;criticalPoints(i,l).jacobi_distance_D];
% 
%        b_g = [b_g; smoothing_constraint(norm(criticalPoints(i,l).roc_A),d_stop,d_influence) .* max((criticalPoints(i,l).jacobi_dist_max_A * (criticalPoints(i,l).jointAngles_critical_A)'),0) ...
%            ; smoothing_constraint(norm(criticalPoints(i,l).roc_D),d_stop,d_influence) .* max((criticalPoints(i,l).jacobi_dist_max_D * (criticalPoints(i,l).jointAngles_critical_D)'),0)]; 
%         %b_g = [b_g; smoothing_constraint(criticalPoints(i,l).roc_D,d_stop,d_influence).* max((criticalPoints(i,l).jacobi_dist_max_D * criticalPoints(i,l).jointAngles_critical_D),0)]; 
% 
% 
%     end
% end 

% % %For speed preallocating 

%maximum number of entries possible
% J_g = zeros(3*2*length(obstacles)*length(linesegments),number_of_joints);
% b_g = zeros(3*2*length(obstacles)*length(linesegments),1);

% The maximum number of entries is defined as:
% here 3 comes from the row size of result of linesegments(i).jacobi_distance (Jx,Jy ,Jz).
% 2 comes from two  possible cases  jacobi_distance_A and  jacobi_distance_D

% Define maximum sizes based on potential maximum entries
maxEntries = 3 * 2 * length(obstacles) * length(linesegments);


% Preallocate arrays
J_g_calculate = zeros(maxEntries, number_of_joints);
b_g_calculate = zeros(maxEntries, 1);


% Counter to keep track of the number of filled entries
J_counter = 0;
b_counter = 0;
for l = 1:length(obstacles)
    for i = 1:length(linesegments)
        % Concatenate the Jacobians if they are not empty
        if ~any(isnan(criticalPoints(i,l).jacobi_distance_A))
            J_g_calculate(J_counter + (1:3), :) = criticalPoints(i,l).jacobi_distance_A;
            J_counter = J_counter + 3;
        end

        if ~any(isnan(criticalPoints(i,l).jacobi_distance_D))
            J_g_calculate(J_counter + (1:3), :) = criticalPoints(i,l).jacobi_distance_D;
            J_counter = J_counter + 3;
        end

        % Compute b_g_calculate elements
        if ~any(isnan(criticalPoints(i,l).roc_A))
            smoothing_value = smoothing_constraint(norm(criticalPoints(i,l).roc_A), d_stop, d_influence);
            b_g_calculate(b_counter + (1:3)) = smoothing_value .* max((criticalPoints(i,l).jacobi_dist_max_A * (criticalPoints(i,l).jointAngles_critical_A)'),0);
            b_counter = b_counter + 3;
        end

        if ~any(isnan(criticalPoints(i,l).roc_D))
            smoothing_value = smoothing_constraint(norm(criticalPoints(i,l).roc_D), d_stop, d_influence);
            b_g_calculate(b_counter + (1:3)) = smoothing_value .* max((criticalPoints(i,l).jacobi_dist_max_D * (criticalPoints(i,l).jointAngles_critical_D)'),0);
            b_counter = b_counter + 3;
        end
    end
end

% Trim the J_g_calculate and b_g_calculate matrices to the actual number of filled entries
J_g = J_g_calculate(1:J_counter, :);
b_g = b_g_calculate(1:b_counter);

== matlab function simulation_file/Manual INVERSE KINEMATICS BlOCK/MATLAB Function1 ==
  data: obstacles output Bus: <object name>
function obstacles = initObstacles()
    % Define the obstacle struct array
% Use an enum or integer to represent the obstacle type for efficiency
persistent obstacles_bus

if isempty(obstacles_bus)
OBSTACLE_SPHERE = 1;
OBSTACLE_CYLINDER = 2;
OBSTACLE_BOX = 3;

obstacle_sphere_1 = struct(...
    'type', OBSTACLE_SPHERE, ...               
    'center', [0, 0.15, 0.8], ...
    'dimensions', [0.05, 0.05, 0.05], ... 
    'orientation', [1, 0, 0, 0], ... 
    'axis', NaN ...        
);

obstacle_sphere_2 = struct(...
    'type', OBSTACLE_SPHERE, ...               
    'center', [0, -0.7, 0.8], ...
    'dimensions', [0.05, 0.05, 0.1], ... 
    'orientation', NaN, ... 
    'axis', NaN ...        
);
obstacles_bus = [obstacle_sphere_1 obstacle_sphere_2];
end 
%obstacles = [obstacle_sphere_1];
    % Add more obstacles if necessary

    Simulink.Bus.createObject(obstacles);
end

== matlab function simulation_file/Add_noise ==
  settings: updateMethod=DISCRETE
  data: joint_vector input; noisy_joint_vector output; noise_min input; noise_max input
function noisy_joint_vector = add_noise(joint_vector,noise_min,noise_max)


% Define the range of the uniform noise
% noise_min = -0.005;
% noise_max = 0.005;

% Generate uniform noise with the same size as the joint vector
noise = noise_min + (noise_max - noise_min) * rand(size(joint_vector));

% Add the noise to the original joint vector
noisy_joint_vector = joint_vector + noise;
end

== matlab function simulation_file/Trajectory Generation/Rotation Trajectory/MATLAB Function ==
  data: t input; hasChanged output; waypointTimes input; segIdx output
function [hasChanged,segIdx] = getTrajIdx(t,waypointTimes)

% Initialize previous index
persistent prevIdx
if isempty(prevIdx)
    prevIdx = 0;
end

% Find the trajectory segment index
segIndices = find(t>=waypointTimes);

% Limit the index value to the number of times minus one
% (This addresses the final time case)
segIdx = min(segIndices(end),numel(waypointTimes)-1);

% Determine whether the index has changed from the previous time step
if prevIdx == segIdx
    hasChanged = false;
else
    hasChanged = true;
    prevIdx = segIdx;
end

end

== matlab function simulation_file/Trajectory Generation/Rotation Trajectory/Extract Trajectory Segment/MATLAB Function1 ==
  data: segIdx input; q0 output; waypointTimes input; orientations input; qf output; timeInterval output
function [q0, qf, timeInterval] = createRotationTrajSegment(segIdx,waypointTimes,orientations)

% Extract the time interval, initial, and final quaternions for the segment
timeInterval = waypointTimes(segIdx:segIdx+1);
q0 = eul2quat(orientations(:,segIdx)');
qf = eul2quat(orientations(:,segIdx+1)');

end
